simulink model "traffic_light_control_moore"  (R2020b)
settings: Solver=VariableStepAuto  StartTime=0.0  StopTime=10.0  RelTol=1e-3
settings Model: Creator=Vrunda M Balgi  LastModifiedBy=Vrunda M Balgi

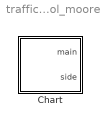
== system traffic_light_control_moore ==
  Chart : Stateflow chart  TreatAsAtomicUnit=on

== stateflow chart traffic_light_control_moore/Chart ==
  state FirstState
    main = GREEN;
    side = RED;
  state SecondState
    main = YELLOW;
    side = RED;
  state ThirdState
    main = RED;
    side = RED;
  state SixthState
    main = RED;
    side = RED;
  state FifthState
    main = RED;
    side = YELLOW;;
  state FourthState
    main = RED;
    side = GREEN;
  (default) -> FirstState
  FirstState -> SecondState
  SecondState -> ThirdState
  SixthState -> FirstState
  ThirdState -> FourthState
  FifthState -> SixthState
  FourthState -> FifthState
  data: GREEN constant double =3; YELLOW constant double =2; RED constant double =1; main output; side output
